simulink model "GS_model"  (R2018b)
settings: Solver=ode5  StartTime=0.0  StopTime=SimuStopTime  FixedStep=T_Simu  RelTol=1e-3
InitFcn:
  | Initial
undefined symbols (not defined in the file or in its folder): Aba10, Aba20, aeroCIP2006_S, aeroCIP2006_X, aeroCIP2006_Y, Agl0, Ass_kS, Ass_n1, Ass_n2, Ass_n3, Ass_n4, Ass_Noise, Ass_R, Ass_Resolution, Ass_TmOrder, AssA_Fix_Abs, AssB_Fix_Abs, AssC_Fix_Abs, AssD_Fix_Abs, AssE_Fix_Aps, AssF_Fix_Aps, C, c_max, c_min, Cd, CenterOfFigNX, CenterOfFigNY, CenterOfFigNZ, CenterOfFigP1, CenterOfFigP2, CenterOfFigPX, CenterOfFigPY, CenterOfFigPZ, Cmu, Crou, DEG2RAD, DiscIntNeverNeededParam, Eg_Dir, Eg_F, Eg_PrepareTime, Eg_r_L_L, Fw_Abf, Fw_Hmax, Fw_J, Fw_Spd0, Fw_Tmax, git_hash_BaseLine, git_hash_Project, Gnss_Noise_Pos, Gnss_Noise_Vel, Gnss_PropgationTime, GyroA_Fix_Abg, GyroA_Noise, GyroB_Fix_Abg, GyroB_Noise, GyroC_Fix_Abg, GyroC_Noise, GyroD_Fix_Abg, GyroD_Noise, h ... (+94)
libraries: simulink x308, sharedutil x46, aerolibutil x37, sharedtransform x31, vrlib x14, aerolibgravity2 x2
(part 15 of 20)

== system GS_model/Subsystem2/Subsystem/Sensor/Gyro/GyroAModel/GyroErrSet/GyroErrSet/GyroErrSet_Wave ==
  w_in : Inport
  ErrSet : Inport  Port=2
  Add : Sum  Inputs=|++
  Add1 : Sum  Inputs=|++
  Add2 : Sum  Inputs=|++
  Compare To Zero : simulink/Logic and Bit Operations/Compare To Zero  relop===  OutDataTypeStr=boolean
  Compare To Zero1 : simulink/Logic and Bit Operations/Compare To Zero  relop===  OutDataTypeStr=boolean
  Compare To Zero2 : simulink/Logic and Bit Operations/Compare To Zero  relop===  OutDataTypeStr=boolean
  Constant : Constant
  Constant1 : Constant  Value=2
  Constant2 : Constant  Value=3
  Demux : Demux  Outputs=3
  Demux1 : Demux  Outputs=3
  Logical Operator : Logic  Operator=OR  AllPortsSameDT=off  OutDataTypeStr=boolean
  Logical Operator1 : Logic  Operator=OR  AllPortsSameDT=off  OutDataTypeStr=boolean
  Logical Operator2 : Logic  Operator=OR  AllPortsSameDT=off  OutDataTypeStr=boolean
  Mux : Mux  Inputs=3
  Product : Product
  Product1 : Product
  Product2 : Product
  Relational Operator1 : RelationalOperator  Operator===  OutDataTypeStr=boolean  RndMeth=Simplest
  Relational Operator2 : RelationalOperator  Operator===  OutDataTypeStr=boolean  RndMeth=Simplest
  Relational Operator5 : RelationalOperator  Operator===  OutDataTypeStr=boolean  RndMeth=Simplest
  Switch1 : Switch  Criteria=u2 > Threshold  Threshold=0.5
  Switch2 : Switch  Criteria=u2 > Threshold  Threshold=0.5
  Switch3 : Switch  Criteria=u2 > Threshold  Threshold=0.5
  Triggered Subsystem1 : Subsystem  TreatAsAtomicUnit=on
  Triggered Subsystem2 : Subsystem  TreatAsAtomicUnit=on
  Triggered Subsystem8 : Subsystem  TreatAsAtomicUnit=on
  WaveSet : SignalGenerator  WaveForm=square  Amplitude=1*DEG2RAD
  w_out : Outport
  wires:
  Product2/1 -> Add2/1
  Product1/1 -> Add1/1
  Product/1 -> Add/1
  w_in/1 -> Demux/1
  Triggered Subsystem1/1(Out1) -> Switch1/2
  Triggered Subsystem8/1(Out1) -> Switch3/2
  WaveSet/1 -> Product/1, Product1/1, Product2/1
  Switch2/1 -> Mux/3
  Triggered Subsystem2/1(Out1) -> Switch2/2
  Demux1/3 -> Product/2, Product1/2, Product2/2  "Coff"
  ErrSet/1 -> Demux1/1
  Switch1/1 -> Mux/2
  Add/1 -> Switch3/1
  Demux/3 -> Add2/2, Switch2/3
  Switch3/1 -> Mux/1
  Demux1/2 -> Triggered Subsystem8/1(In1), Triggered Subsystem1/1(In1), Triggered Subsystem2/1(In1)  "Switch"
  Add1/1 -> Switch1/1
  Mux/1 -> w_out/1
  Add2/1 -> Switch2/1
  Demux/2 -> Switch1/3, Add1/2
  Demux/1 -> Switch3/3, Add/2
  Relational Operator5/1 -> Logical Operator/2
  Logical Operator/1 -> Triggered Subsystem8/Enable
  Compare To Zero/1 -> Logical Operator/1
  Constant/1 -> Relational Operator5/2
  Constant1/1 -> Relational Operator1/2
  Compare To Zero1/1 -> Logical Operator1/1
  Logical Operator1/1 -> Triggered Subsystem1/Enable
  Relational Operator1/1 -> Logical Operator1/2
  Demux1/1 -> Compare To Zero/1, Relational Operator5/1, Compare To Zero1/1, Relational Operator1/1, Compare To Zero2/1, Relational Operator2/1
  Relational Operator2/1 -> Logical Operator2/2
  Logical Operator2/1 -> Triggered Subsystem2/Enable
  Compare To Zero2/1 -> Logical Operator2/1
  Constant2/1 -> Relational Operator2/2

== system GS_model/Subsystem2/Subsystem/Sensor/Gyro/GyroAModel/GyroErrSet/GyroErrSet/GyroErrSet_WildValue ==
  w_in : Inport
  ErrSwitch : Inport  Port=2
  Compare To Zero : simulink/Logic and Bit Operations/Compare To Zero  relop===  OutDataTypeStr=boolean
  Compare To Zero1 : simulink/Logic and Bit Operations/Compare To Zero  relop===  OutDataTypeStr=boolean
  Compare To Zero2 : simulink/Logic and Bit Operations/Compare To Zero  relop===  OutDataTypeStr=boolean
  Constant3 : Constant  Value=8.5*DEG2RAD
  Constant4 : Constant
  Constant5 : Constant  Value=2
  Constant6 : Constant  Value=3
  Demux : Demux  Outputs=3
  Demux1 : Demux  Outputs=2
  Logical Operator : Logic  Operator=OR  AllPortsSameDT=off  OutDataTypeStr=boolean
  Logical Operator1 : Logic  Operator=OR  AllPortsSameDT=off  OutDataTypeStr=boolean
  Logical Operator2 : Logic  Operator=OR  AllPortsSameDT=off  OutDataTypeStr=boolean
  Mux : Mux  Inputs=3
  Relational Operator3 : RelationalOperator  Operator===  OutDataTypeStr=boolean  RndMeth=Simplest
  Relational Operator4 : RelationalOperator  Operator===  OutDataTypeStr=boolean  RndMeth=Simplest
  Relational Operator5 : RelationalOperator  Operator===  OutDataTypeStr=boolean  RndMeth=Simplest
  Switch1 : Switch  Criteria=u2 > Threshold  Threshold=0.5
  Switch2 : Switch  Criteria=u2 > Threshold  Threshold=0.5
  Switch3 : Switch  Criteria=u2 > Threshold  Threshold=0.5
  Triggered Subsystem1 : Subsystem  TreatAsAtomicUnit=on
  Triggered Subsystem2 : Subsystem  TreatAsAtomicUnit=on
  Triggered Subsystem8 : Subsystem  TreatAsAtomicUnit=on
  w_out : Outport
  wires:
  Mux/1 -> w_out/1
  Logical Operator2/1 -> Triggered Subsystem2/Enable
  Logical Operator1/1 -> Triggered Subsystem1/Enable
  Triggered Subsystem8/1(Out1) -> Switch1/2
  Logical Operator/1 -> Triggered Subsystem8/Enable
  Triggered Subsystem2/1(Out1) -> Switch3/2
  Switch3/1 -> Mux/3
  Demux/3 -> Switch3/3
  Triggered Subsystem1/1(Out1) -> Switch2/2
  Switch2/1 -> Mux/2
  Demux/2 -> Switch2/3
  Demux/1 -> Switch1/3
  ErrSwitch/1 -> Demux1/1
  Switch1/1 -> Mux/1
  w_in/1 -> Demux/1
  Constant3/1 -> Switch3/1, Switch2/1, Switch1/1
  Compare To Zero/1 -> Logical Operator/1
  Compare To Zero1/1 -> Logical Operator1/1
  Compare To Zero2/1 -> Logical Operator2/1
  Relational Operator4/1 -> Logical Operator2/2
  Constant6/1 -> Relational Operator4/2
  Demux1/1 -> Relational Operator5/1, Compare To Zero1/1, Compare To Zero2/1, Relational Operator4/1, Relational Operator3/1, Compare To Zero/1
  Constant4/1 -> Relational Operator5/2
  Relational Operator3/1 -> Logical Operator1/2
  Relational Operator5/1 -> Logical Operator/2
  Constant5/1 -> Relational Operator3/2
  Demux1/2 -> Triggered Subsystem2/1(In1), Triggered Subsystem1/1(In1), Triggered Subsystem8/1(In1)

== system GS_model/Subsystem2/Subsystem/Sensor/Gyro/GyroBModel/GyroErrSet/GyroErrSet/GyroErrSet_Constant ==
  w_in : Inport
  ErrSwitch : Inport  Port=2
  Compare To Zero : simulink/Logic and Bit Operations/Compare To Zero  relop===  OutDataTypeStr=boolean
  Compare To Zero1 : simulink/Logic and Bit Operations/Compare To Zero  relop===  OutDataTypeStr=boolean
  Compare To Zero2 : simulink/Logic and Bit Operations/Compare To Zero  relop===  OutDataTypeStr=boolean
  Constant : Constant
  Constant1 : Constant  Value=2
  Constant2 : Constant  Value=3
  Demux : Demux  Outputs=3
  Demux1 : Demux  Outputs=2
  Logical Operator : Logic  Operator=OR  AllPortsSameDT=off  OutDataTypeStr=boolean
  Logical Operator1 : Logic  Operator=OR  AllPortsSameDT=off  OutDataTypeStr=boolean
  Logical Operator2 : Logic  Operator=OR  AllPortsSameDT=off  OutDataTypeStr=boolean
  Memory : Memory
  Memory1 : Memory
  Memory2 : Memory
  Mux : Mux  Inputs=3
  Relational Operator1 : RelationalOperator  Operator===  OutDataTypeStr=boolean  RndMeth=Simplest
  Relational Operator2 : RelationalOperator  Operator===  OutDataTypeStr=boolean  RndMeth=Simplest
  Relational Operator9 : RelationalOperator  Operator===  OutDataTypeStr=boolean  RndMeth=Simplest
  Switch1 : Switch  Criteria=u2 > Threshold  Threshold=0.5
  Switch2 : Switch  Criteria=u2 > Threshold  Threshold=0.5
  Switch3 : Switch  Criteria=u2 > Threshold  Threshold=0.5
  Triggered Subsystem1 : Subsystem  TreatAsAtomicUnit=on
  Triggered Subsystem2 : Subsystem  TreatAsAtomicUnit=on
  Triggered Subsystem8 : Subsystem  TreatAsAtomicUnit=on
  w_out : Outport
  wires:
  w_in/1 -> Demux/1
  Switch1/1 -> Memory/1, Mux/1
  Memory/1 -> Switch1/1
  ErrSwitch/1 -> Demux1/1
  Demux/1 -> Switch1/3
  Demux/2 -> Switch2/3
  Memory1/1 -> Switch2/1
  Switch2/1 -> Mux/2, Memory1/1
  Triggered Subsystem1/1(Out1) -> Switch2/2
  Demux/3 -> Switch3/3
  Memory2/1 -> Switch3/1
  Switch3/1 -> Mux/3, Memory2/1
  Triggered Subsystem2/1(Out1) -> Switch3/2
  Constant/1 -> Relational Operator9/2
  Triggered Subsystem8/1(Out1) -> Switch1/2
  Constant1/1 -> Relational Operator1/2
  Demux1/1 -> Relational Operator9/1, Compare To Zero1/1, Compare To Zero2/1, Relational Operator2/1, Relational Operator1/1, Compare To Zero/1
  Demux1/2 -> Triggered Subsystem8/1(In1), Triggered Subsystem2/1(In1), Triggered Subsystem1/1(In1)
  Constant2/1 -> Relational Operator2/2
  Mux/1 -> w_out/1
  Logical Operator/1 -> Triggered Subsystem8/Enable
  Relational Operator9/1 -> Logical Operator/2
  Compare To Zero/1 -> Logical Operator/1
  Relational Operator1/1 -> Logical Operator1/2
  Logical Operator1/1 -> Triggered Subsystem1/Enable
  Compare To Zero1/1 -> Logical Operator1/1
  Relational Operator2/1 -> Logical Operator2/2
  Compare To Zero2/1 -> Logical Operator2/1
  Logical Operator2/1 -> Triggered Subsystem2/Enable

== system GS_model/Subsystem2/Subsystem/Sensor/Gyro/GyroBModel/GyroErrSet/GyroErrSet/GyroErrSet_Jump ==
  w_in : Inport
  ErrSet : Inport  Port=2
  Add : Sum  Inputs=|++
  Add1 : Sum  Inputs=|++
  Add2 : Sum  Inputs=|++
  Compare To Zero : simulink/Logic and Bit Operations/Compare To Zero  relop===  OutDataTypeStr=boolean
  Compare To Zero1 : simulink/Logic and Bit Operations/Compare To Zero  relop===  OutDataTypeStr=boolean
  Compare To Zero2 : simulink/Logic and Bit Operations/Compare To Zero  relop===  OutDataTypeStr=boolean
  Constant : Constant
  Constant1 : Constant  Value=2
  Constant2 : Constant  Value=3
  Demux : Demux  Outputs=3
  Demux1 : Demux
  JumpSet : Constant  Value=1*DEG2RAD
  Logical Operator : Logic  Operator=OR  AllPortsSameDT=off  OutDataTypeStr=boolean
  Logical Operator1 : Logic  Operator=OR  AllPortsSameDT=off  OutDataTypeStr=boolean
  Logical Operator2 : Logic  Operator=OR  AllPortsSameDT=off  OutDataTypeStr=boolean
  Mux : Mux  Inputs=3
  Product : Product
  Product1 : Product
  Product2 : Product
  Relational Operator1 : RelationalOperator  Operator===  OutDataTypeStr=boolean  RndMeth=Simplest
  Relational Operator2 : RelationalOperator  Operator===  OutDataTypeStr=boolean  RndMeth=Simplest
  Relational Operator5 : RelationalOperator  Operator===  OutDataTypeStr=boolean  RndMeth=Simplest
  Switch1 : Switch  Criteria=u2 > Threshold  Threshold=0.5
  Switch2 : Switch  Criteria=u2 > Threshold  Threshold=0.5
  Switch3 : Switch  Criteria=u2 > Threshold  Threshold=0.5
  Terminator : Terminator
  Triggered Subsystem1 : Subsystem  TreatAsAtomicUnit=on
  Triggered Subsystem2 : Subsystem  TreatAsAtomicUnit=on
  Triggered Subsystem8 : Subsystem  TreatAsAtomicUnit=on
  w_out : Outport
  wires:
  Demux/1 -> Add/2, Switch3/3
  Demux/2 -> Add1/2, Switch1/3
  Add2/1 -> Switch2/1
  Mux/1 -> w_out/1
  Add1/1 -> Switch1/1
  Demux1/2 -> Triggered Subsystem8/1(In1), Triggered Subsystem1/1(In1), Triggered Subsystem2/1(In1)  "Switch"
  Switch3/1 -> Mux/1
  Demux/3 -> Switch2/3, Add2/2
  Add/1 -> Switch3/1
  Demux1/3 -> Terminator/1  "Period"
  Switch1/1 -> Mux/2
  ErrSet/1 -> Demux1/1
  Demux1/4 -> Product2/2, Product1/2, Product/2  "Coff"
  Constant1/1 -> Relational Operator1/2
  Triggered Subsystem2/1(Out1) -> Switch2/2
  Switch2/1 -> Mux/3
  JumpSet/1 -> Product2/1, Product1/1, Product/1
  Triggered Subsystem8/1(Out1) -> Switch3/2
  Constant/1 -> Relational Operator5/2
  Triggered Subsystem1/1(Out1) -> Switch1/2
  w_in/1 -> Demux/1
  Product/1 -> Add/1
  Product1/1 -> Add1/1
  Product2/1 -> Add2/1
  Relational Operator5/1 -> Logical Operator/2
  Logical Operator/1 -> Triggered Subsystem8/Enable
  Compare To Zero/1 -> Logical Operator/1
  Compare To Zero1/1 -> Logical Operator1/1
  Logical Operator1/1 -> Triggered Subsystem1/Enable
  Relational Operator1/1 -> Logical Operator1/2
  Demux1/1 -> Compare To Zero1/1, Relational Operator1/1, Compare To Zero2/1, Relational Operator2/1, Relational Operator5/1, Compare To Zero/1
  Relational Operator2/1 -> Logical Operator2/2
  Logical Operator2/1 -> Triggered Subsystem2/Enable
  Compare To Zero2/1 -> Logical Operator2/1
  Constant2/1 -> Relational Operator2/2

== system GS_model/Subsystem2/Subsystem/Sensor/Gyro/GyroBModel/GyroErrSet/GyroErrSet/GyroErrSet_Wave ==
  w_in : Inport
  ErrSet : Inport  Port=2
  Add : Sum  Inputs=|++
  Add1 : Sum  Inputs=|++
  Add2 : Sum  Inputs=|++
  Compare To Zero : simulink/Logic and Bit Operations/Compare To Zero  relop===  OutDataTypeStr=boolean
  Compare To Zero1 : simulink/Logic and Bit Operations/Compare To Zero  relop===  OutDataTypeStr=boolean
  Compare To Zero2 : simulink/Logic and Bit Operations/Compare To Zero  relop===  OutDataTypeStr=boolean
  Constant : Constant
  Constant1 : Constant  Value=2
  Constant2 : Constant  Value=3
  Demux : Demux  Outputs=3
  Demux1 : Demux  Outputs=3
  Logical Operator : Logic  Operator=OR  AllPortsSameDT=off  OutDataTypeStr=boolean
  Logical Operator1 : Logic  Operator=OR  AllPortsSameDT=off  OutDataTypeStr=boolean
  Logical Operator2 : Logic  Operator=OR  AllPortsSameDT=off  OutDataTypeStr=boolean
  Mux : Mux  Inputs=3
  Product : Product
  Product1 : Product
  Product2 : Product
  Relational Operator1 : RelationalOperator  Operator===  OutDataTypeStr=boolean  RndMeth=Simplest
  Relational Operator2 : RelationalOperator  Operator===  OutDataTypeStr=boolean  RndMeth=Simplest
  Relational Operator5 : RelationalOperator  Operator===  OutDataTypeStr=boolean  RndMeth=Simplest
  Switch1 : Switch  Criteria=u2 > Threshold  Threshold=0.5
  Switch2 : Switch  Criteria=u2 > Threshold  Threshold=0.5
  Switch3 : Switch  Criteria=u2 > Threshold  Threshold=0.5
  Triggered Subsystem1 : Subsystem  TreatAsAtomicUnit=on
  Triggered Subsystem2 : Subsystem  TreatAsAtomicUnit=on
  Triggered Subsystem8 : Subsystem  TreatAsAtomicUnit=on
  WaveSet : SignalGenerator  WaveForm=square  Amplitude=1*DEG2RAD
  w_out : Outport
  wires:
  Product2/1 -> Add2/1
  Product1/1 -> Add1/1
  Product/1 -> Add/1
  w_in/1 -> Demux/1
  Triggered Subsystem1/1(Out1) -> Switch1/2
  Triggered Subsystem8/1(Out1) -> Switch3/2
  WaveSet/1 -> Product/1, Product1/1, Product2/1
  Switch2/1 -> Mux/3
  Triggered Subsystem2/1(Out1) -> Switch2/2
  Demux1/3 -> Product/2, Product1/2, Product2/2  "Coff"
  ErrSet/1 -> Demux1/1
  Switch1/1 -> Mux/2
  Add/1 -> Switch3/1
  Demux/3 -> Add2/2, Switch2/3
  Switch3/1 -> Mux/1
  Demux1/2 -> Triggered Subsystem8/1(In1), Triggered Subsystem1/1(In1), Triggered Subsystem2/1(In1)  "Switch"
  Add1/1 -> Switch1/1
  Mux/1 -> w_out/1
  Add2/1 -> Switch2/1
  Demux/2 -> Switch1/3, Add1/2
  Demux/1 -> Switch3/3, Add/2
  Relational Operator5/1 -> Logical Operator/2
  Logical Operator/1 -> Triggered Subsystem8/Enable
  Compare To Zero/1 -> Logical Operator/1
  Constant/1 -> Relational Operator5/2
  Constant1/1 -> Relational Operator1/2
  Compare To Zero1/1 -> Logical Operator1/1
  Logical Operator1/1 -> Triggered Subsystem1/Enable
  Relational Operator1/1 -> Logical Operator1/2
  Demux1/1 -> Compare To Zero/1, Relational Operator5/1, Compare To Zero1/1, Relational Operator1/1, Compare To Zero2/1, Relational Operator2/1
  Relational Operator2/1 -> Logical Operator2/2
  Logical Operator2/1 -> Triggered Subsystem2/Enable
  Compare To Zero2/1 -> Logical Operator2/1
  Constant2/1 -> Relational Operator2/2

== system GS_model/Subsystem2/Subsystem/Sensor/Gyro/GyroBModel/GyroErrSet/GyroErrSet/GyroErrSet_WildValue ==
  w_in : Inport
  ErrSwitch : Inport  Port=2
  Compare To Zero : simulink/Logic and Bit Operations/Compare To Zero  relop===  OutDataTypeStr=boolean
  Compare To Zero1 : simulink/Logic and Bit Operations/Compare To Zero  relop===  OutDataTypeStr=boolean
  Compare To Zero2 : simulink/Logic and Bit Operations/Compare To Zero  relop===  OutDataTypeStr=boolean
  Constant3 : Constant  Value=8.5*DEG2RAD
  Constant4 : Constant
  Constant5 : Constant  Value=2
  Constant6 : Constant  Value=3
  Demux : Demux  Outputs=3
  Demux1 : Demux  Outputs=2
  Logical Operator : Logic  Operator=OR  AllPortsSameDT=off  OutDataTypeStr=boolean
  Logical Operator1 : Logic  Operator=OR  AllPortsSameDT=off  OutDataTypeStr=boolean
  Logical Operator2 : Logic  Operator=OR  AllPortsSameDT=off  OutDataTypeStr=boolean
  Mux : Mux  Inputs=3
  Relational Operator3 : RelationalOperator  Operator===  OutDataTypeStr=boolean  RndMeth=Simplest
  Relational Operator4 : RelationalOperator  Operator===  OutDataTypeStr=boolean  RndMeth=Simplest
  Relational Operator5 : RelationalOperator  Operator===  OutDataTypeStr=boolean  RndMeth=Simplest
  Switch1 : Switch  Criteria=u2 > Threshold  Threshold=0.5
  Switch2 : Switch  Criteria=u2 > Threshold  Threshold=0.5
  Switch3 : Switch  Criteria=u2 > Threshold  Threshold=0.5
  Triggered Subsystem1 : Subsystem  TreatAsAtomicUnit=on
  Triggered Subsystem2 : Subsystem  TreatAsAtomicUnit=on
  Triggered Subsystem8 : Subsystem  TreatAsAtomicUnit=on
  w_out : Outport
  wires:
  Mux/1 -> w_out/1
  Logical Operator2/1 -> Triggered Subsystem2/Enable
  Logical Operator1/1 -> Triggered Subsystem1/Enable
  Triggered Subsystem8/1(Out1) -> Switch1/2
  Logical Operator/1 -> Triggered Subsystem8/Enable
  Triggered Subsystem2/1(Out1) -> Switch3/2
  Switch3/1 -> Mux/3
  Demux/3 -> Switch3/3
  Triggered Subsystem1/1(Out1) -> Switch2/2
  Switch2/1 -> Mux/2
  Demux/2 -> Switch2/3
  Demux/1 -> Switch1/3
  ErrSwitch/1 -> Demux1/1
  Switch1/1 -> Mux/1
  w_in/1 -> Demux/1
  Constant3/1 -> Switch3/1, Switch2/1, Switch1/1
  Compare To Zero/1 -> Logical Operator/1
  Compare To Zero1/1 -> Logical Operator1/1
  Compare To Zero2/1 -> Logical Operator2/1
  Relational Operator4/1 -> Logical Operator2/2
  Constant6/1 -> Relational Operator4/2
  Demux1/1 -> Relational Operator5/1, Compare To Zero1/1, Compare To Zero2/1, Relational Operator4/1, Relational Operator3/1, Compare To Zero/1
  Constant4/1 -> Relational Operator5/2
  Relational Operator3/1 -> Logical Operator1/2
  Relational Operator5/1 -> Logical Operator/2
  Constant5/1 -> Relational Operator3/2
  Demux1/2 -> Triggered Subsystem2/1(In1), Triggered Subsystem1/1(In1), Triggered Subsystem8/1(In1)

== system GS_model/Subsystem2/Subsystem/Sensor/Gyro/GyroCModel/GyroErrSet/GyroErrSet/GyroErrSet_Constant ==
  w_in : Inport
  ErrSwitch : Inport  Port=2
  Compare To Zero : simulink/Logic and Bit Operations/Compare To Zero  relop===  OutDataTypeStr=boolean
  Compare To Zero1 : simulink/Logic and Bit Operations/Compare To Zero  relop===  OutDataTypeStr=boolean
  Compare To Zero2 : simulink/Logic and Bit Operations/Compare To Zero  relop===  OutDataTypeStr=boolean
  Constant : Constant
  Constant1 : Constant  Value=2
  Constant2 : Constant  Value=3
  Demux : Demux  Outputs=3
  Demux1 : Demux  Outputs=2
  Logical Operator : Logic  Operator=OR  AllPortsSameDT=off  OutDataTypeStr=boolean
  Logical Operator1 : Logic  Operator=OR  AllPortsSameDT=off  OutDataTypeStr=boolean
  Logical Operator2 : Logic  Operator=OR  AllPortsSameDT=off  OutDataTypeStr=boolean
  Memory : Memory
  Memory1 : Memory
  Memory2 : Memory
  Mux : Mux  Inputs=3
  Relational Operator1 : RelationalOperator  Operator===  OutDataTypeStr=boolean  RndMeth=Simplest
  Relational Operator2 : RelationalOperator  Operator===  OutDataTypeStr=boolean  RndMeth=Simplest
  Relational Operator9 : RelationalOperator  Operator===  OutDataTypeStr=boolean  RndMeth=Simplest
  Switch1 : Switch  Criteria=u2 > Threshold  Threshold=0.5
  Switch2 : Switch  Criteria=u2 > Threshold  Threshold=0.5
  Switch3 : Switch  Criteria=u2 > Threshold  Threshold=0.5
  Triggered Subsystem1 : Subsystem  TreatAsAtomicUnit=on
  Triggered Subsystem2 : Subsystem  TreatAsAtomicUnit=on
  Triggered Subsystem8 : Subsystem  TreatAsAtomicUnit=on
  w_out : Outport
  wires:
  w_in/1 -> Demux/1
  Switch1/1 -> Memory/1, Mux/1
  Memory/1 -> Switch1/1
  ErrSwitch/1 -> Demux1/1
  Demux/1 -> Switch1/3
  Demux/2 -> Switch2/3
  Memory1/1 -> Switch2/1
  Switch2/1 -> Mux/2, Memory1/1
  Triggered Subsystem1/1(Out1) -> Switch2/2
  Demux/3 -> Switch3/3
  Memory2/1 -> Switch3/1
  Switch3/1 -> Mux/3, Memory2/1
  Triggered Subsystem2/1(Out1) -> Switch3/2
  Constant/1 -> Relational Operator9/2
  Triggered Subsystem8/1(Out1) -> Switch1/2
  Constant1/1 -> Relational Operator1/2
  Demux1/1 -> Relational Operator9/1, Compare To Zero1/1, Compare To Zero2/1, Relational Operator2/1, Relational Operator1/1, Compare To Zero/1
  Demux1/2 -> Triggered Subsystem8/1(In1), Triggered Subsystem2/1(In1), Triggered Subsystem1/1(In1)
  Constant2/1 -> Relational Operator2/2
  Mux/1 -> w_out/1
  Logical Operator/1 -> Triggered Subsystem8/Enable
  Relational Operator9/1 -> Logical Operator/2
  Compare To Zero/1 -> Logical Operator/1
  Relational Operator1/1 -> Logical Operator1/2
  Logical Operator1/1 -> Triggered Subsystem1/Enable
  Compare To Zero1/1 -> Logical Operator1/1
  Relational Operator2/1 -> Logical Operator2/2
  Compare To Zero2/1 -> Logical Operator2/1
  Logical Operator2/1 -> Triggered Subsystem2/Enable

== system GS_model/Subsystem2/Subsystem/Sensor/Gyro/GyroCModel/GyroErrSet/GyroErrSet/GyroErrSet_Jump ==
  w_in : Inport
  ErrSet : Inport  Port=2
  Add : Sum  Inputs=|++
  Add1 : Sum  Inputs=|++
  Add2 : Sum  Inputs=|++
  Compare To Zero : simulink/Logic and Bit Operations/Compare To Zero  relop===  OutDataTypeStr=boolean
  Compare To Zero1 : simulink/Logic and Bit Operations/Compare To Zero  relop===  OutDataTypeStr=boolean
  Compare To Zero2 : simulink/Logic and Bit Operations/Compare To Zero  relop===  OutDataTypeStr=boolean
  Constant : Constant
  Constant1 : Constant  Value=2
  Constant2 : Constant  Value=3
  Demux : Demux  Outputs=3
  Demux1 : Demux
  JumpSet : Constant  Value=1*DEG2RAD
  Logical Operator : Logic  Operator=OR  AllPortsSameDT=off  OutDataTypeStr=boolean
  Logical Operator1 : Logic  Operator=OR  AllPortsSameDT=off  OutDataTypeStr=boolean
  Logical Operator2 : Logic  Operator=OR  AllPortsSameDT=off  OutDataTypeStr=boolean
  Mux : Mux  Inputs=3
  Product : Product
  Product1 : Product
  Product2 : Product
  Relational Operator1 : RelationalOperator  Operator===  OutDataTypeStr=boolean  RndMeth=Simplest
  Relational Operator2 : RelationalOperator  Operator===  OutDataTypeStr=boolean  RndMeth=Simplest
  Relational Operator5 : RelationalOperator  Operator===  OutDataTypeStr=boolean  RndMeth=Simplest
  Switch1 : Switch  Criteria=u2 > Threshold  Threshold=0.5
  Switch2 : Switch  Criteria=u2 > Threshold  Threshold=0.5
  Switch3 : Switch  Criteria=u2 > Threshold  Threshold=0.5
  Terminator : Terminator
  Triggered Subsystem1 : Subsystem  TreatAsAtomicUnit=on
  Triggered Subsystem2 : Subsystem  TreatAsAtomicUnit=on
  Triggered Subsystem8 : Subsystem  TreatAsAtomicUnit=on
  w_out : Outport
  wires:
  Demux/1 -> Add/2, Switch3/3
  Demux/2 -> Add1/2, Switch1/3
  Add2/1 -> Switch2/1
  Mux/1 -> w_out/1
  Add1/1 -> Switch1/1
  Demux1/2 -> Triggered Subsystem8/1(In1), Triggered Subsystem1/1(In1), Triggered Subsystem2/1(In1)  "Switch"
  Switch3/1 -> Mux/1
  Demux/3 -> Switch2/3, Add2/2
  Add/1 -> Switch3/1
  Demux1/3 -> Terminator/1  "Period"
  Switch1/1 -> Mux/2
  ErrSet/1 -> Demux1/1
  Demux1/4 -> Product2/2, Product1/2, Product/2  "Coff"
  Constant1/1 -> Relational Operator1/2
  Triggered Subsystem2/1(Out1) -> Switch2/2
  Switch2/1 -> Mux/3
  JumpSet/1 -> Product2/1, Product1/1, Product/1
  Triggered Subsystem8/1(Out1) -> Switch3/2
  Constant/1 -> Relational Operator5/2
  Triggered Subsystem1/1(Out1) -> Switch1/2
  w_in/1 -> Demux/1
  Product/1 -> Add/1
  Product1/1 -> Add1/1
  Product2/1 -> Add2/1
  Relational Operator5/1 -> Logical Operator/2
  Logical Operator/1 -> Triggered Subsystem8/Enable
  Compare To Zero/1 -> Logical Operator/1
  Compare To Zero1/1 -> Logical Operator1/1
  Logical Operator1/1 -> Triggered Subsystem1/Enable
  Relational Operator1/1 -> Logical Operator1/2
  Demux1/1 -> Compare To Zero1/1, Relational Operator1/1, Compare To Zero2/1, Relational Operator2/1, Relational Operator5/1, Compare To Zero/1
  Relational Operator2/1 -> Logical Operator2/2
  Logical Operator2/1 -> Triggered Subsystem2/Enable
  Compare To Zero2/1 -> Logical Operator2/1
  Constant2/1 -> Relational Operator2/2

== system GS_model/Subsystem2/Subsystem/Sensor/Gyro/GyroCModel/GyroErrSet/GyroErrSet/GyroErrSet_Wave ==
  w_in : Inport
  ErrSet : Inport  Port=2
  Add : Sum  Inputs=|++
  Add1 : Sum  Inputs=|++
  Add2 : Sum  Inputs=|++
  Compare To Zero : simulink/Logic and Bit Operations/Compare To Zero  relop===  OutDataTypeStr=boolean
  Compare To Zero1 : simulink/Logic and Bit Operations/Compare To Zero  relop===  OutDataTypeStr=boolean
  Compare To Zero2 : simulink/Logic and Bit Operations/Compare To Zero  relop===  OutDataTypeStr=boolean
  Constant : Constant
  Constant1 : Constant  Value=2
  Constant2 : Constant  Value=3
  Demux : Demux  Outputs=3
  Demux1 : Demux  Outputs=3
  Logical Operator : Logic  Operator=OR  AllPortsSameDT=off  OutDataTypeStr=boolean
  Logical Operator1 : Logic  Operator=OR  AllPortsSameDT=off  OutDataTypeStr=boolean
  Logical Operator2 : Logic  Operator=OR  AllPortsSameDT=off  OutDataTypeStr=boolean
  Mux : Mux  Inputs=3
  Product : Product
  Product1 : Product
  Product2 : Product
  Relational Operator1 : RelationalOperator  Operator===  OutDataTypeStr=boolean  RndMeth=Simplest
  Relational Operator2 : RelationalOperator  Operator===  OutDataTypeStr=boolean  RndMeth=Simplest
  Relational Operator5 : RelationalOperator  Operator===  OutDataTypeStr=boolean  RndMeth=Simplest
  Switch1 : Switch  Criteria=u2 > Threshold  Threshold=0.5
  Switch2 : Switch  Criteria=u2 > Threshold  Threshold=0.5
  Switch3 : Switch  Criteria=u2 > Threshold  Threshold=0.5
  Triggered Subsystem1 : Subsystem  TreatAsAtomicUnit=on
  Triggered Subsystem2 : Subsystem  TreatAsAtomicUnit=on
  Triggered Subsystem8 : Subsystem  TreatAsAtomicUnit=on
  WaveSet : SignalGenerator  WaveForm=square  Amplitude=1*DEG2RAD
  w_out : Outport
  wires:
  Product2/1 -> Add2/1
  Product1/1 -> Add1/1
  Product/1 -> Add/1
  w_in/1 -> Demux/1
  Triggered Subsystem1/1(Out1) -> Switch1/2
  Triggered Subsystem8/1(Out1) -> Switch3/2
  WaveSet/1 -> Product/1, Product1/1, Product2/1
  Switch2/1 -> Mux/3
  Triggered Subsystem2/1(Out1) -> Switch2/2
  Demux1/3 -> Product/2, Product1/2, Product2/2  "Coff"
  ErrSet/1 -> Demux1/1
  Switch1/1 -> Mux/2
  Add/1 -> Switch3/1
  Demux/3 -> Add2/2, Switch2/3
  Switch3/1 -> Mux/1
  Demux1/2 -> Triggered Subsystem8/1(In1), Triggered Subsystem1/1(In1), Triggered Subsystem2/1(In1)  "Switch"
  Add1/1 -> Switch1/1
  Mux/1 -> w_out/1
  Add2/1 -> Switch2/1
  Demux/2 -> Switch1/3, Add1/2
  Demux/1 -> Switch3/3, Add/2
  Relational Operator5/1 -> Logical Operator/2
  Logical Operator/1 -> Triggered Subsystem8/Enable
  Compare To Zero/1 -> Logical Operator/1
  Constant/1 -> Relational Operator5/2
  Constant1/1 -> Relational Operator1/2
  Compare To Zero1/1 -> Logical Operator1/1
  Logical Operator1/1 -> Triggered Subsystem1/Enable
  Relational Operator1/1 -> Logical Operator1/2
  Demux1/1 -> Compare To Zero/1, Relational Operator5/1, Compare To Zero1/1, Relational Operator1/1, Compare To Zero2/1, Relational Operator2/1
  Relational Operator2/1 -> Logical Operator2/2
  Logical Operator2/1 -> Triggered Subsystem2/Enable
  Compare To Zero2/1 -> Logical Operator2/1
  Constant2/1 -> Relational Operator2/2

== system GS_model/Subsystem2/Subsystem/Sensor/Gyro/GyroCModel/GyroErrSet/GyroErrSet/GyroErrSet_WildValue ==
  w_in : Inport
  ErrSwitch : Inport  Port=2
  Compare To Zero : simulink/Logic and Bit Operations/Compare To Zero  relop===  OutDataTypeStr=boolean
  Compare To Zero1 : simulink/Logic and Bit Operations/Compare To Zero  relop===  OutDataTypeStr=boolean
  Compare To Zero2 : simulink/Logic and Bit Operations/Compare To Zero  relop===  OutDataTypeStr=boolean
  Constant3 : Constant  Value=8.5*DEG2RAD
  Constant4 : Constant
  Constant5 : Constant  Value=2
  Constant6 : Constant  Value=3
  Demux : Demux  Outputs=3
  Demux1 : Demux  Outputs=2
  Logical Operator : Logic  Operator=OR  AllPortsSameDT=off  OutDataTypeStr=boolean
  Logical Operator1 : Logic  Operator=OR  AllPortsSameDT=off  OutDataTypeStr=boolean
  Logical Operator2 : Logic  Operator=OR  AllPortsSameDT=off  OutDataTypeStr=boolean
  Mux : Mux  Inputs=3
  Relational Operator3 : RelationalOperator  Operator===  OutDataTypeStr=boolean  RndMeth=Simplest
  Relational Operator4 : RelationalOperator  Operator===  OutDataTypeStr=boolean  RndMeth=Simplest
  Relational Operator5 : RelationalOperator  Operator===  OutDataTypeStr=boolean  RndMeth=Simplest
  Switch1 : Switch  Criteria=u2 > Threshold  Threshold=0.5
  Switch2 : Switch  Criteria=u2 > Threshold  Threshold=0.5
  Switch3 : Switch  Criteria=u2 > Threshold  Threshold=0.5
  Triggered Subsystem1 : Subsystem  TreatAsAtomicUnit=on
  Triggered Subsystem2 : Subsystem  TreatAsAtomicUnit=on
  Triggered Subsystem8 : Subsystem  TreatAsAtomicUnit=on
  w_out : Outport
  wires:
  Mux/1 -> w_out/1
  Logical Operator2/1 -> Triggered Subsystem2/Enable
  Logical Operator1/1 -> Triggered Subsystem1/Enable
  Triggered Subsystem8/1(Out1) -> Switch1/2
  Logical Operator/1 -> Triggered Subsystem8/Enable
  Triggered Subsystem2/1(Out1) -> Switch3/2
  Switch3/1 -> Mux/3
  Demux/3 -> Switch3/3
  Triggered Subsystem1/1(Out1) -> Switch2/2
  Switch2/1 -> Mux/2
  Demux/2 -> Switch2/3
  Demux/1 -> Switch1/3
  ErrSwitch/1 -> Demux1/1
  Switch1/1 -> Mux/1
  w_in/1 -> Demux/1
  Constant3/1 -> Switch3/1, Switch2/1, Switch1/1
  Compare To Zero/1 -> Logical Operator/1
  Compare To Zero1/1 -> Logical Operator1/1
  Compare To Zero2/1 -> Logical Operator2/1
  Relational Operator4/1 -> Logical Operator2/2
  Constant6/1 -> Relational Operator4/2
  Demux1/1 -> Relational Operator5/1, Compare To Zero1/1, Compare To Zero2/1, Relational Operator4/1, Relational Operator3/1, Compare To Zero/1
  Constant4/1 -> Relational Operator5/2
  Relational Operator3/1 -> Logical Operator1/2
  Relational Operator5/1 -> Logical Operator/2
  Constant5/1 -> Relational Operator3/2
  Demux1/2 -> Triggered Subsystem2/1(In1), Triggered Subsystem1/1(In1), Triggered Subsystem8/1(In1)

== system GS_model/Subsystem2/Subsystem/Sensor/Gyro/GyroDModel/GyroErrSet/GyroErrSet/GyroErrSet_Constant ==
  w_in : Inport
  ErrSwitch : Inport  Port=2
  Compare To Zero : simulink/Logic and Bit Operations/Compare To Zero  relop===  OutDataTypeStr=boolean
  Compare To Zero1 : simulink/Logic and Bit Operations/Compare To Zero  relop===  OutDataTypeStr=boolean
  Compare To Zero2 : simulink/Logic and Bit Operations/Compare To Zero  relop===  OutDataTypeStr=boolean
  Constant : Constant
  Constant1 : Constant  Value=2
  Constant2 : Constant  Value=3
  Demux : Demux  Outputs=3
  Demux1 : Demux  Outputs=2
  Logical Operator : Logic  Operator=OR  AllPortsSameDT=off  OutDataTypeStr=boolean
  Logical Operator1 : Logic  Operator=OR  AllPortsSameDT=off  OutDataTypeStr=boolean
  Logical Operator2 : Logic  Operator=OR  AllPortsSameDT=off  OutDataTypeStr=boolean
  Memory : Memory
  Memory1 : Memory
  Memory2 : Memory
  Mux : Mux  Inputs=3
  Relational Operator1 : RelationalOperator  Operator===  OutDataTypeStr=boolean  RndMeth=Simplest
  Relational Operator2 : RelationalOperator  Operator===  OutDataTypeStr=boolean  RndMeth=Simplest
  Relational Operator9 : RelationalOperator  Operator===  OutDataTypeStr=boolean  RndMeth=Simplest
  Switch1 : Switch  Criteria=u2 > Threshold  Threshold=0.5
  Switch2 : Switch  Criteria=u2 > Threshold  Threshold=0.5
  Switch3 : Switch  Criteria=u2 > Threshold  Threshold=0.5
  Triggered Subsystem1 : Subsystem  TreatAsAtomicUnit=on
  Triggered Subsystem2 : Subsystem  TreatAsAtomicUnit=on
  Triggered Subsystem8 : Subsystem  TreatAsAtomicUnit=on
  w_out : Outport
  wires:
  w_in/1 -> Demux/1
  Switch1/1 -> Memory/1, Mux/1
  Memory/1 -> Switch1/1
  ErrSwitch/1 -> Demux1/1
  Demux/1 -> Switch1/3
  Demux/2 -> Switch2/3
  Memory1/1 -> Switch2/1
  Switch2/1 -> Mux/2, Memory1/1
  Triggered Subsystem1/1(Out1) -> Switch2/2
  Demux/3 -> Switch3/3
  Memory2/1 -> Switch3/1
  Switch3/1 -> Mux/3, Memory2/1
  Triggered Subsystem2/1(Out1) -> Switch3/2
  Constant/1 -> Relational Operator9/2
  Triggered Subsystem8/1(Out1) -> Switch1/2
  Constant1/1 -> Relational Operator1/2
  Demux1/1 -> Relational Operator9/1, Compare To Zero1/1, Compare To Zero2/1, Relational Operator2/1, Relational Operator1/1, Compare To Zero/1
  Demux1/2 -> Triggered Subsystem8/1(In1), Triggered Subsystem2/1(In1), Triggered Subsystem1/1(In1)
  Constant2/1 -> Relational Operator2/2
  Mux/1 -> w_out/1
  Logical Operator/1 -> Triggered Subsystem8/Enable
  Relational Operator9/1 -> Logical Operator/2
  Compare To Zero/1 -> Logical Operator/1
  Relational Operator1/1 -> Logical Operator1/2
  Logical Operator1/1 -> Triggered Subsystem1/Enable
  Compare To Zero1/1 -> Logical Operator1/1
  Relational Operator2/1 -> Logical Operator2/2
  Compare To Zero2/1 -> Logical Operator2/1
  Logical Operator2/1 -> Triggered Subsystem2/Enable

== system GS_model/Subsystem2/Subsystem/Sensor/Gyro/GyroDModel/GyroErrSet/GyroErrSet/GyroErrSet_Jump ==
  w_in : Inport
  ErrSet : Inport  Port=2
  Add : Sum  Inputs=|++
  Add1 : Sum  Inputs=|++
  Add2 : Sum  Inputs=|++
  Compare To Zero : simulink/Logic and Bit Operations/Compare To Zero  relop===  OutDataTypeStr=boolean
  Compare To Zero1 : simulink/Logic and Bit Operations/Compare To Zero  relop===  OutDataTypeStr=boolean
  Compare To Zero2 : simulink/Logic and Bit Operations/Compare To Zero  relop===  OutDataTypeStr=boolean
  Constant : Constant
  Constant1 : Constant  Value=2
  Constant2 : Constant  Value=3
  Demux : Demux  Outputs=3
  Demux1 : Demux
  JumpSet : Constant  Value=1*DEG2RAD
  Logical Operator : Logic  Operator=OR  AllPortsSameDT=off  OutDataTypeStr=boolean
  Logical Operator1 : Logic  Operator=OR  AllPortsSameDT=off  OutDataTypeStr=boolean
  Logical Operator2 : Logic  Operator=OR  AllPortsSameDT=off  OutDataTypeStr=boolean
  Mux : Mux  Inputs=3
  Product : Product
  Product1 : Product
  Product2 : Product
  Relational Operator1 : RelationalOperator  Operator===  OutDataTypeStr=boolean  RndMeth=Simplest
  Relational Operator2 : RelationalOperator  Operator===  OutDataTypeStr=boolean  RndMeth=Simplest
  Relational Operator5 : RelationalOperator  Operator===  OutDataTypeStr=boolean  RndMeth=Simplest
  Switch1 : Switch  Criteria=u2 > Threshold  Threshold=0.5
  Switch2 : Switch  Criteria=u2 > Threshold  Threshold=0.5
  Switch3 : Switch  Criteria=u2 > Threshold  Threshold=0.5
  Terminator : Terminator
  Triggered Subsystem1 : Subsystem  TreatAsAtomicUnit=on
  Triggered Subsystem2 : Subsystem  TreatAsAtomicUnit=on
  Triggered Subsystem8 : Subsystem  TreatAsAtomicUnit=on
  w_out : Outport
  wires:
  Demux/1 -> Add/2, Switch3/3
  Demux/2 -> Add1/2, Switch1/3
  Add2/1 -> Switch2/1
  Mux/1 -> w_out/1
  Add1/1 -> Switch1/1
  Demux1/2 -> Triggered Subsystem8/1(In1), Triggered Subsystem1/1(In1), Triggered Subsystem2/1(In1)  "Switch"
  Switch3/1 -> Mux/1
  Demux/3 -> Switch2/3, Add2/2
  Add/1 -> Switch3/1
  Demux1/3 -> Terminator/1  "Period"
  Switch1/1 -> Mux/2
  ErrSet/1 -> Demux1/1
  Demux1/4 -> Product2/2, Product1/2, Product/2  "Coff"
  Constant1/1 -> Relational Operator1/2
  Triggered Subsystem2/1(Out1) -> Switch2/2
  Switch2/1 -> Mux/3
  JumpSet/1 -> Product2/1, Product1/1, Product/1
  Triggered Subsystem8/1(Out1) -> Switch3/2
  Constant/1 -> Relational Operator5/2
  Triggered Subsystem1/1(Out1) -> Switch1/2
  w_in/1 -> Demux/1
  Product/1 -> Add/1
  Product1/1 -> Add1/1
  Product2/1 -> Add2/1
  Relational Operator5/1 -> Logical Operator/2
  Logical Operator/1 -> Triggered Subsystem8/Enable
  Compare To Zero/1 -> Logical Operator/1
  Compare To Zero1/1 -> Logical Operator1/1
  Logical Operator1/1 -> Triggered Subsystem1/Enable
  Relational Operator1/1 -> Logical Operator1/2
  Demux1/1 -> Compare To Zero1/1, Relational Operator1/1, Compare To Zero2/1, Relational Operator2/1, Relational Operator5/1, Compare To Zero/1
  Relational Operator2/1 -> Logical Operator2/2
  Logical Operator2/1 -> Triggered Subsystem2/Enable
  Compare To Zero2/1 -> Logical Operator2/1
  Constant2/1 -> Relational Operator2/2

== system GS_model/Subsystem2/Subsystem/Sensor/Gyro/GyroDModel/GyroErrSet/GyroErrSet/GyroErrSet_Wave ==
  w_in : Inport
  ErrSet : Inport  Port=2
  Add : Sum  Inputs=|++
  Add1 : Sum  Inputs=|++
  Add2 : Sum  Inputs=|++
  Compare To Zero : simulink/Logic and Bit Operations/Compare To Zero  relop===  OutDataTypeStr=boolean
  Compare To Zero1 : simulink/Logic and Bit Operations/Compare To Zero  relop===  OutDataTypeStr=boolean
  Compare To Zero2 : simulink/Logic and Bit Operations/Compare To Zero  relop===  OutDataTypeStr=boolean
  Constant : Constant
  Constant1 : Constant  Value=2
  Constant2 : Constant  Value=3
  Demux : Demux  Outputs=3
  Demux1 : Demux  Outputs=3
  Logical Operator : Logic  Operator=OR  AllPortsSameDT=off  OutDataTypeStr=boolean
  Logical Operator1 : Logic  Operator=OR  AllPortsSameDT=off  OutDataTypeStr=boolean
  Logical Operator2 : Logic  Operator=OR  AllPortsSameDT=off  OutDataTypeStr=boolean
  Mux : Mux  Inputs=3
  Product : Product
  Product1 : Product
  Product2 : Product
  Relational Operator1 : RelationalOperator  Operator===  OutDataTypeStr=boolean  RndMeth=Simplest
  Relational Operator2 : RelationalOperator  Operator===  OutDataTypeStr=boolean  RndMeth=Simplest
  Relational Operator5 : RelationalOperator  Operator===  OutDataTypeStr=boolean  RndMeth=Simplest
  Switch1 : Switch  Criteria=u2 > Threshold  Threshold=0.5
  Switch2 : Switch  Criteria=u2 > Threshold  Threshold=0.5
  Switch3 : Switch  Criteria=u2 > Threshold  Threshold=0.5
  Triggered Subsystem1 : Subsystem  TreatAsAtomicUnit=on
  Triggered Subsystem2 : Subsystem  TreatAsAtomicUnit=on
  Triggered Subsystem8 : Subsystem  TreatAsAtomicUnit=on
  WaveSet : SignalGenerator  WaveForm=square  Amplitude=1*DEG2RAD
  w_out : Outport
  wires:
  Product2/1 -> Add2/1
  Product1/1 -> Add1/1
  Product/1 -> Add/1
  w_in/1 -> Demux/1
  Triggered Subsystem1/1(Out1) -> Switch1/2
  Triggered Subsystem8/1(Out1) -> Switch3/2
  WaveSet/1 -> Product/1, Product1/1, Product2/1
  Switch2/1 -> Mux/3
  Triggered Subsystem2/1(Out1) -> Switch2/2
  Demux1/3 -> Product/2, Product1/2, Product2/2  "Coff"
  ErrSet/1 -> Demux1/1
  Switch1/1 -> Mux/2
  Add/1 -> Switch3/1
  Demux/3 -> Add2/2, Switch2/3
  Switch3/1 -> Mux/1
  Demux1/2 -> Triggered Subsystem8/1(In1), Triggered Subsystem1/1(In1), Triggered Subsystem2/1(In1)  "Switch"
  Add1/1 -> Switch1/1
  Mux/1 -> w_out/1
  Add2/1 -> Switch2/1
  Demux/2 -> Switch1/3, Add1/2
  Demux/1 -> Switch3/3, Add/2
  Relational Operator5/1 -> Logical Operator/2
  Logical Operator/1 -> Triggered Subsystem8/Enable
  Compare To Zero/1 -> Logical Operator/1
  Constant/1 -> Relational Operator5/2
  Constant1/1 -> Relational Operator1/2
  Compare To Zero1/1 -> Logical Operator1/1
  Logical Operator1/1 -> Triggered Subsystem1/Enable
  Relational Operator1/1 -> Logical Operator1/2
  Demux1/1 -> Compare To Zero/1, Relational Operator5/1, Compare To Zero1/1, Relational Operator1/1, Compare To Zero2/1, Relational Operator2/1
  Relational Operator2/1 -> Logical Operator2/2
  Logical Operator2/1 -> Triggered Subsystem2/Enable
  Compare To Zero2/1 -> Logical Operator2/1
  Constant2/1 -> Relational Operator2/2

== system GS_model/Subsystem2/Subsystem/Sensor/Gyro/GyroDModel/GyroErrSet/GyroErrSet/GyroErrSet_WildValue ==
  w_in : Inport
  ErrSwitch : Inport  Port=2
  Compare To Zero : simulink/Logic and Bit Operations/Compare To Zero  relop===  OutDataTypeStr=boolean
  Compare To Zero1 : simulink/Logic and Bit Operations/Compare To Zero  relop===  OutDataTypeStr=boolean
  Compare To Zero2 : simulink/Logic and Bit Operations/Compare To Zero  relop===  OutDataTypeStr=boolean
  Constant3 : Constant  Value=8.5*DEG2RAD
  Constant4 : Constant
  Constant5 : Constant  Value=2
  Constant6 : Constant  Value=3
  Demux : Demux  Outputs=3
  Demux1 : Demux  Outputs=2
  Logical Operator : Logic  Operator=OR  AllPortsSameDT=off  OutDataTypeStr=boolean
  Logical Operator1 : Logic  Operator=OR  AllPortsSameDT=off  OutDataTypeStr=boolean
  Logical Operator2 : Logic  Operator=OR  AllPortsSameDT=off  OutDataTypeStr=boolean
  Mux : Mux  Inputs=3
  Relational Operator3 : RelationalOperator  Operator===  OutDataTypeStr=boolean  RndMeth=Simplest
  Relational Operator4 : RelationalOperator  Operator===  OutDataTypeStr=boolean  RndMeth=Simplest
  Relational Operator5 : RelationalOperator  Operator===  OutDataTypeStr=boolean  RndMeth=Simplest
  Switch1 : Switch  Criteria=u2 > Threshold  Threshold=0.5
  Switch2 : Switch  Criteria=u2 > Threshold  Threshold=0.5
  Switch3 : Switch  Criteria=u2 > Threshold  Threshold=0.5
  Triggered Subsystem1 : Subsystem  TreatAsAtomicUnit=on
  Triggered Subsystem2 : Subsystem  TreatAsAtomicUnit=on
  Triggered Subsystem8 : Subsystem  TreatAsAtomicUnit=on
  w_out : Outport
  wires:
  Mux/1 -> w_out/1
  Logical Operator2/1 -> Triggered Subsystem2/Enable
  Logical Operator1/1 -> Triggered Subsystem1/Enable
  Triggered Subsystem8/1(Out1) -> Switch1/2
  Logical Operator/1 -> Triggered Subsystem8/Enable
  Triggered Subsystem2/1(Out1) -> Switch3/2
  Switch3/1 -> Mux/3
  Demux/3 -> Switch3/3
  Triggered Subsystem1/1(Out1) -> Switch2/2
  Switch2/1 -> Mux/2
  Demux/2 -> Switch2/3
  Demux/1 -> Switch1/3
  ErrSwitch/1 -> Demux1/1
  Switch1/1 -> Mux/1
  w_in/1 -> Demux/1
  Constant3/1 -> Switch3/1, Switch2/1, Switch1/1
  Compare To Zero/1 -> Logical Operator/1
  Compare To Zero1/1 -> Logical Operator1/1
  Compare To Zero2/1 -> Logical Operator2/1
  Relational Operator4/1 -> Logical Operator2/2
  Constant6/1 -> Relational Operator4/2
  Demux1/1 -> Relational Operator5/1, Compare To Zero1/1, Compare To Zero2/1, Relational Operator4/1, Relational Operator3/1, Compare To Zero/1
  Constant4/1 -> Relational Operator5/2
  Relational Operator3/1 -> Logical Operator1/2
  Relational Operator5/1 -> Logical Operator/2
  Constant5/1 -> Relational Operator3/2
  Demux1/2 -> Triggered Subsystem2/1(In1), Triggered Subsystem1/1(In1), Triggered Subsystem8/1(In1)

== system GS_model/Subsystem2/Subsystem/Sensor/Magnetometer/MmModel1/Mm_ErrSet/MmErrSet/MmErrSet_Constant ==
  Mm_in : Inport
  ErrSwitch : Inport  Port=2
  Constant1 : Constant  Value=2
  Constant2 : Constant  Value=3
  Constant3 : Constant
  Demux : Demux  Outputs=3
  MmAxisXErrSet_Constant : Subsystem
  MmAxisXErrSet_Constant1 : Subsystem
  MmAxisXErrSet_Constant2 : Subsystem
  Mux : Mux  Inputs=3
  Mm_out : Outport
  wires:
  Mm_in/1 -> Demux/1
  Mux/1 -> Mm_out/1
  Demux/1 -> MmAxisXErrSet_Constant/1(MmAxis_in)
  ErrSwitch/1 -> MmAxisXErrSet_Constant2/2(ErrSwitch), MmAxisXErrSet_Constant1/2(ErrSwitch), MmAxisXErrSet_Constant/2(ErrSwitch)
  Constant3/1 -> MmAxisXErrSet_Constant/3(MmAxis_Num)
  MmAxisXErrSet_Constant/1(MmAxis_out) -> Mux/1
  Constant1/1 -> MmAxisXErrSet_Constant1/3(MmAxis_Num)
  Constant2/1 -> MmAxisXErrSet_Constant2/3(MmAxis_Num)
  Demux/2 -> MmAxisXErrSet_Constant1/1(MmAxis_in)
  Demux/3 -> MmAxisXErrSet_Constant2/1(MmAxis_in)
  MmAxisXErrSet_Constant1/1(MmAxis_out) -> Mux/2
  MmAxisXErrSet_Constant2/1(MmAxis_out) -> Mux/3

== system GS_model/Subsystem2/Subsystem/Sensor/Magnetometer/MmModel1/Mm_ErrSet/MmErrSet/MmErrSet_Jump ==
  Mm_in : Inport
  ErrSet : Inport  Port=2
  Constant3 : Constant
  Constant4 : Constant  Value=2
  Constant5 : Constant  Value=3
  Demux : Demux  Outputs=3
  JumpSet : Constant  Value=0.2
  MmAxisXErrSet_Jump : Subsystem
  MmAxisXErrSet_Jump1 : Subsystem
  MmAxisXErrSet_Jump2 : Subsystem
  Mux : Mux  Inputs=3
  Mm_out : Outport
  wires:
  Mux/1 -> Mm_out/1
  Mm_in/1 -> Demux/1
  Demux/1 -> MmAxisXErrSet_Jump/1(MmAxis_in)
  ErrSet/1 -> MmAxisXErrSet_Jump2/2(ErrSet), MmAxisXErrSet_Jump1/2(ErrSet), MmAxisXErrSet_Jump/2(ErrSet)
  Constant3/1 -> MmAxisXErrSet_Jump/3(MmAxis_Num)
  JumpSet/1 -> MmAxisXErrSet_Jump2/4(MmAxis_JumpSet), MmAxisXErrSet_Jump1/4(MmAxis_JumpSet), MmAxisXErrSet_Jump/4(MmAxis_JumpSet)
  Constant4/1 -> MmAxisXErrSet_Jump1/3(MmAxis_Num)
  Constant5/1 -> MmAxisXErrSet_Jump2/3(MmAxis_Num)
  Demux/2 -> MmAxisXErrSet_Jump1/1(MmAxis_in)
  Demux/3 -> MmAxisXErrSet_Jump2/1(MmAxis_in)
  MmAxisXErrSet_Jump1/1(MmAxis_out) -> Mux/2
  MmAxisXErrSet_Jump/1(MmAxis_out) -> Mux/1
  MmAxisXErrSet_Jump2/1(MmAxis_out) -> Mux/3

== system GS_model/Subsystem2/Subsystem/Sensor/Magnetometer/MmModel1/Mm_ErrSet/MmErrSet/MmErrSet_Wave ==
  Mm_in : Inport
  ErrSet : Inport  Port=2
  Constant1 : Constant  Value=2
  Constant2 : Constant  Value=3
  Constant3 : Constant
  Demux : Demux  Outputs=3
  MmAxisXErrSet_Wave : Subsystem
  MmAxisXErrSet_Wave1 : Subsystem
  MmAxisXErrSet_Wave2 : Subsystem
  Mux : Mux  Inputs=3
  WaveSet : SignalGenerator  WaveForm=square  Amplitude=0.2
  Mm_out : Outport
  wires:
  Mm_in/1 -> Demux/1
  Mux/1 -> Mm_out/1
  Demux/1 -> MmAxisXErrSet_Wave/1(MmAxis_in)
  ErrSet/1 -> MmAxisXErrSet_Wave2/2(ErrSet), MmAxisXErrSet_Wave1/2(ErrSet), MmAxisXErrSet_Wave/2(ErrSet)
  Constant3/1 -> MmAxisXErrSet_Wave/3(MmAxis_Num)
  WaveSet/1 -> MmAxisXErrSet_Wave2/4(MmAxis_WaveSet), MmAxisXErrSet_Wave1/4(MmAxis_WaveSet), MmAxisXErrSet_Wave/4(MmAxis_WaveSet)
  MmAxisXErrSet_Wave1/1(MmAxis_out) -> Mux/2
  MmAxisXErrSet_Wave/1(MmAxis_out) -> Mux/1
  MmAxisXErrSet_Wave2/1(MmAxis_out) -> Mux/3
  Constant1/1 -> MmAxisXErrSet_Wave1/3(MmAxis_Num)
  Constant2/1 -> MmAxisXErrSet_Wave2/3(MmAxis_Num)
  Demux/2 -> MmAxisXErrSet_Wave1/1(MmAxis_in)
  Demux/3 -> MmAxisXErrSet_Wave2/1(MmAxis_in)

== system GS_model/Subsystem2/Subsystem/Sensor/Magnetometer/MmModel1/Mm_ErrSet/MmErrSet/MmErrSet_WildValue ==
  Mm_in : Inport
  ErrSwitch : Inport  Port=2
  Constant : Constant
  Constant1 : Constant  Value=2
  Constant2 : Constant  Value=3
  Demux : Demux  Outputs=3
  MmAxisXErrSet_WildValue : Subsystem
  MmAxisXErrSet_WildValue1 : Subsystem
  MmAxisXErrSet_WildValue2 : Subsystem
  Mux : Mux  Inputs=3
  WildValue : Constant  Value=2
  Mm_out : Outport
  wires:
  Mux/1 -> Mm_out/1
  Mm_in/1 -> Demux/1
  Constant/1 -> MmAxisXErrSet_WildValue/3(MmAxis_Num)
  WildValue/1 -> MmAxisXErrSet_WildValue2/4(MmAxis_WildValue), MmAxisXErrSet_WildValue1/4(MmAxis_WildValue), MmAxisXErrSet_WildValue/4(MmAxis_WildValue)
  Demux/1 -> MmAxisXErrSet_WildValue/1(MmAxis_in)
  ErrSwitch/1 -> MmAxisXErrSet_WildValue2/2(ErrSwitch), MmAxisXErrSet_WildValue1/2(ErrSwitch), MmAxisXErrSet_WildValue/2(ErrSwitch)
  MmAxisXErrSet_WildValue/1(MmAxis_out) -> Mux/1
  Constant1/1 -> MmAxisXErrSet_WildValue1/3(MmAxis_Num)
  Constant2/1 -> MmAxisXErrSet_WildValue2/3(MmAxis_Num)
  Demux/2 -> MmAxisXErrSet_WildValue1/1(MmAxis_in)
  Demux/3 -> MmAxisXErrSet_WildValue2/1(MmAxis_in)
  MmAxisXErrSet_WildValue1/1(MmAxis_out) -> Mux/2
  MmAxisXErrSet_WildValue2/1(MmAxis_out) -> Mux/3

== system GS_model/Subsystem2/Subsystem/Sensor/Magnetometer/MmModel2/Mm_ErrSet/MmErrSet/MmErrSet_Constant ==
  Mm_in : Inport
  ErrSwitch : Inport  Port=2
  Constant1 : Constant  Value=2
  Constant2 : Constant  Value=3
  Constant3 : Constant
  Demux : Demux  Outputs=3
  MmAxisXErrSet_Constant : Subsystem
  MmAxisXErrSet_Constant1 : Subsystem
  MmAxisXErrSet_Constant2 : Subsystem
  Mux : Mux  Inputs=3
  Mm_out : Outport
  wires:
  MmAxisXErrSet_Constant2/1(MmAxis_out) -> Mux/3
  MmAxisXErrSet_Constant1/1(MmAxis_out) -> Mux/2
  Demux/3 -> MmAxisXErrSet_Constant2/1(MmAxis_in)
  Demux/2 -> MmAxisXErrSet_Constant1/1(MmAxis_in)
  Constant2/1 -> MmAxisXErrSet_Constant2/3(MmAxis_Num)
  Constant1/1 -> MmAxisXErrSet_Constant1/3(MmAxis_Num)
  MmAxisXErrSet_Constant/1(MmAxis_out) -> Mux/1
  Constant3/1 -> MmAxisXErrSet_Constant/3(MmAxis_Num)
  ErrSwitch/1 -> MmAxisXErrSet_Constant/2(ErrSwitch), MmAxisXErrSet_Constant1/2(ErrSwitch), MmAxisXErrSet_Constant2/2(ErrSwitch)
  Demux/1 -> MmAxisXErrSet_Constant/1(MmAxis_in)
  Mux/1 -> Mm_out/1
  Mm_in/1 -> Demux/1

== system GS_model/Subsystem2/Subsystem/Sensor/Magnetometer/MmModel2/Mm_ErrSet/MmErrSet/MmErrSet_Jump ==
  Mm_in : Inport
  ErrSet : Inport  Port=2
  Constant3 : Constant
  Constant4 : Constant  Value=2
  Constant5 : Constant  Value=3
  Demux : Demux  Outputs=3
  JumpSet : Constant  Value=0.2
  MmAxisXErrSet_Jump : Subsystem
  MmAxisXErrSet_Jump1 : Subsystem
  MmAxisXErrSet_Jump2 : Subsystem
  Mux : Mux  Inputs=3
  Mm_out : Outport
  wires:
  MmAxisXErrSet_Jump2/1(MmAxis_out) -> Mux/3
  MmAxisXErrSet_Jump/1(MmAxis_out) -> Mux/1
  MmAxisXErrSet_Jump1/1(MmAxis_out) -> Mux/2
  Demux/3 -> MmAxisXErrSet_Jump2/1(MmAxis_in)
  Demux/2 -> MmAxisXErrSet_Jump1/1(MmAxis_in)
  Constant5/1 -> MmAxisXErrSet_Jump2/3(MmAxis_Num)
  Constant4/1 -> MmAxisXErrSet_Jump1/3(MmAxis_Num)
  JumpSet/1 -> MmAxisXErrSet_Jump/4(MmAxis_JumpSet), MmAxisXErrSet_Jump1/4(MmAxis_JumpSet), MmAxisXErrSet_Jump2/4(MmAxis_JumpSet)
  Constant3/1 -> MmAxisXErrSet_Jump/3(MmAxis_Num)
  ErrSet/1 -> MmAxisXErrSet_Jump/2(ErrSet), MmAxisXErrSet_Jump1/2(ErrSet), MmAxisXErrSet_Jump2/2(ErrSet)
  Demux/1 -> MmAxisXErrSet_Jump/1(MmAxis_in)
  Mm_in/1 -> Demux/1
  Mux/1 -> Mm_out/1
